simulink model "sm_trackV_test_frame_IdlerArm_i2u0r3"  (R2026a)
settings: Solver=VariableStepAuto  AbsTol=1e-3  EnableMultiTasking=on
undefined symbols (not defined in the file): Trac, X, Y, Z
libraries: sm_trackV_lib_belt_underc_elem x5, sm_lib x4, sm_trackV_lib_frame_idlerArm_i2u0l3 x1, nesl_utility x1
Description:
  | Copyright 2024-2026 The MathWorks, Inc.
settings Model: Creator=smiller  LastModifiedBy=smiller
settings DebuggingCC: SubsystemReferenceDiagnosticForUnitTest=warning
settings SimscapeCC: SimscapeNominalValues="[{\"value\":\"1\",\"unit\":\"A\"},{\"value\":\"1\",\"unit\":\"bar\"},{\"value\":\"1\",\"unit\":\"cm^2\"},{\"value\":\"1\",\"unit\":\"cm^3/s\"},{\"value\":\"1\",\"unit\":\"kJ/kg\"},{\"value\":\"1\",\"unit\":\"kW\"},{\"value\":\"1\",\"unit\":\"l\"},{\"value\":\"1\",\"unit\":\"N\"},{\"value\":\"1\",\"unit\":\"N*m\"},{\"value\":\"1\",\"unit\":\"V\"}]"  SimscapeLogSimulationStatistics=on
settings ExplorerConfigSet: InternalSimMechanicsExplorerSettings="<ExplorerConfiguration><canonicalview>default</canonicalview><AnimationSetting><BasePlaybackSpeed>1.0</BasePlaybackSpeed><PlaybackSpeedFactor>1.0</PlaybackSpeedFactor></AnimationSetting><TilePanel><TileInfo><Tiles Columns=\"1\" Count=\"1\" Rows=\"1\"><Column Weight=\"1\"/><Row Weight=\"1\"/><Tile Height=\"1\" Width=\"1\" X=\"0\" Y=\"0\"/></Tiles></TileInfo><SceneInfo><SceneViewer><BGColor><R>1</R><G>1</G><B>1</B></BGColor><Camera><DoPerspective>off</DoPerspective><Position><X>0.754785288464031145</X><Y>-1.88317428009450927</Y><Z>0.0238268327668960112</Z></Position><Center><X>-0.102012532308323189</X><Y>0.0261516749909807</Y><Z>-0.414185312493715541</Z></Center><Up><X>-0.0551998131405338766</X><Y>0.199660102991916943</Y><Z>0.97830916580726579</Z></Up><ViewLimDist>1</ViewLimDist><YLim>1.08093997579067946</YLim><XLim>1.28111404538154594</XLim></Camera></SceneViewer></SceneInfo></TilePanel><MechEditorPanel><Cameras/><GfxPanelCameraMap/><VideoCreator><PlaybackSpeedRatio>1.0</PlaybackSpeedRatio><FrameRate>30</FrameRate><VideoFormat>Motion JPEG AVI</VideoFormat><FrameSize>auto</FrameSize></VideoCreator></MechEditorPanel></ExplorerConfiguration>"

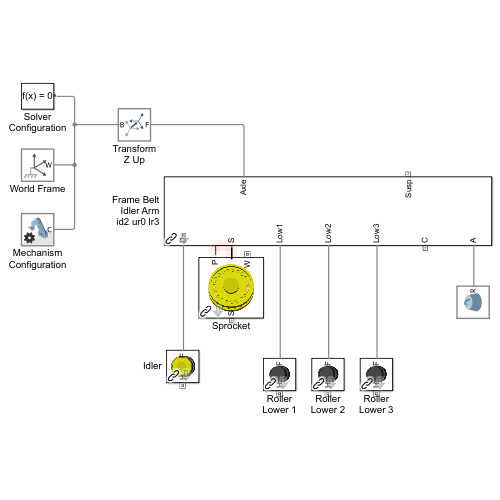
[thumbnail: Simulink's stored preview of the top-level diagram]
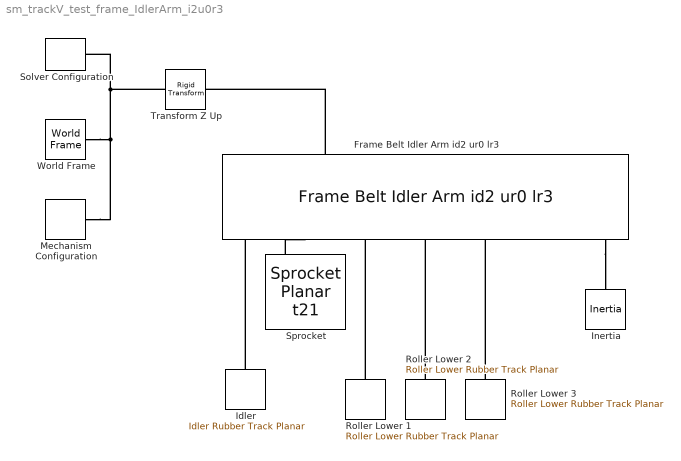
== system sm_trackV_test_frame_IdlerArm_i2u0r3 ==
  Frame Belt Idler Arm id2 ur0 lr3 : sm_trackV_lib_frame_idlerArm_i2u0l3/Frame Belt Idler Arm id2 ur0 lr3  popup_leftOrRight=Right  popup_trackFrame=Revolute  roller_lower_x=Trac.Frame.SprkOffLon.Lower  idlerArm_x=Trac.Frame.SprkOffLon.IdlerArm  idlerFix_x=Trac.Frame.SprkOffLon.IdlerR  tensionC_x=Trac.Frame.SprkOffLon.TensionC  frame_pivot_x=Trac.Frame.SprkOffLon.PivotFra  axle_x=Trac.Frame.SprkOffLon.Axle  roller_lower_y=Trac.Frame.SprkOffVer.Lower  idlerArm_y=Trac.Frame.SprkOffVer.IdlerArm  idlerFix_y=Trac.Frame.SprkOffVer.IdlerR  tensionC_y=Trac.Frame.SprkOffVer.TensionC  frame_pivot_y=Trac.Frame.SprkOffVer.PivotFra  axle_y=Trac.Frame.SprkOffVer.Axle  frame_roller_cg_offset=Trac.Frame.TrackFrame.CG  frame_roller_mass=Trac.Frame.TrackFrame.Mass  frame_roller_moi=Trac.Frame.TrackFrame.MOI  frame_roller_poi=Trac.Frame.TrackFrame.POI  frame_cg_offset=Trac.Frame.SprkFrame.CG  frame_mass=Trac.Frame.SprkFrame.Mass  frame_moi=Trac.Frame.SprkFrame.MOI  frame_poi=Trac.Frame.SprkFrame.POI  frame_susp_offset=Trac.Frame.SuspOffset  roller_frame_pivot_range=Trac.Frame.PivotFra.Range  roller_frame_pivot_k=Trac.Frame.PivotFra.LimitK  roller_frame_pivot_b=Trac.Frame.PivotFra.LimitB  roller_frame_pivot_tw=Trac.Frame.PivotFra.LimitTW
  Idler : sm_trackV_lib_belt_underc_elem/Idler Rubber Track Planar  idler_rad=Trac.IdlerF.rad  idler_len=Trac.IdlerF.len  wheel_clr=Trac.IdlerF.Wheel.clr  rim_rad=Trac.IdlerF.Rim.rad  rim_hub_rad=Trac.IdlerF.Rim.hub_rad  rim_xc=Trac.IdlerF.Rim.rim_xc  idler_rho=Trac.IdlerF.rho  idler_opc=Trac.IdlerF.opc  idler_clr=Trac.IdlerF.clr  idler_axle_rad=Trac.IdlerF.Axle.rad  idler_axle_len=Trac.IdlerF.Axle.len  idler_axle_rho=Trac.IdlerF.Axle.rho  idler_axle_opc=Trac.IdlerF.Axle.opc  idler_axle_clr=Trac.IdlerF.Axle.clr  idler_contgeo_clr=Trac.IdlerF.belt_contact.clr  idler_contgeo_opc=Trac.IdlerF.belt_contact.opc
  Inertia : sm_lib/Body Elements/Inertia  InertiaType=PointMass  Mass=1  MassUnits=kg  CenterOfMass=[0 0 0]  CenterOfMassUnits=m  MomentsOfInertia=[1 1 1]  MomentsOfInertiaUnits=kg*m^2  ProductsOfInertia=[0 0 0]  ProductsOfInertiaUnits=kg*m^2  GraphicType=Marker  MarkerShape=Inertia  MarkerSize=20  GraphicVisPropType=SimpleVisualProperties  GraphicDiffuseColor=[0.5 0.5 0.5]  GraphicOpacity=1.0  GraphicSpecularColor=[0.5 0.5 0.5 1.0]  GraphicAmbientColor=[0.15 0.15 0.15 1.0]  GraphicEmissiveColor=[0.0 0.0 0.0 1.0]  GraphicShininess=75
  Mechanism Configuration : sm_lib/Utilities/Mechanism Configuration  UniformGravity=Constant  GravityVector=[0 0 -9.80665]  GravityVectorUnits=m/s^2  LinearizationDelta=0.001  JointModeTransitionNonlinearIterations=2
  Roller Lower 1 : sm_trackV_lib_belt_underc_elem/Roller Lower Rubber Track Planar  roller_lower_rad=Trac.Roller.Lower.rad  roller_lower_len=Trac.Roller.Lower.len  roller_lower_rho=Trac.Roller.Lower.rho  roller_lower_clr=Trac.Roller.Lower.clr  roller_lower_opc=Trac.Roller.Lower.opc  roller_lower_rim_thk=Trac.Roller.Lower.rim_thk  roller_lower_rim_len=Trac.Roller.Lower.rim_len  roller_lower_axle_rad=Trac.Roller.Lower.Axle.rad  roller_lower_axle_len=Trac.Roller.Lower.Axle.len  roller_lower_axle_rho=Trac.Roller.Lower.Axle.rho  roller_lower_axle_opc=Trac.Roller.Lower.Axle.opc  roller_lower_axle_clr=Trac.Roller.Lower.Axle.clr  roller_lower_contgeo_clr=Trac.Roller.Lower.belt_contact.ptcld.clr  roller_lower_contgeo_opc=Trac.Roller.Lower.belt_contact.ptcld.opc
  Roller Lower 2 : sm_trackV_lib_belt_underc_elem/Roller Lower Rubber Track Planar  roller_lower_rad=Trac.Roller.Lower.rad  roller_lower_len=Trac.Roller.Lower.len  roller_lower_rho=Trac.Roller.Lower.rho  roller_lower_clr=Trac.Roller.Lower.clr  roller_lower_opc=Trac.Roller.Lower.opc  roller_lower_rim_thk=Trac.Roller.Lower.rim_thk  roller_lower_rim_len=Trac.Roller.Lower.rim_len  roller_lower_axle_rad=Trac.Roller.Lower.Axle.rad  roller_lower_axle_len=Trac.Roller.Lower.Axle.len  roller_lower_axle_rho=Trac.Roller.Lower.Axle.rho  roller_lower_axle_opc=Trac.Roller.Lower.Axle.opc  roller_lower_axle_clr=Trac.Roller.Lower.Axle.clr  roller_lower_contgeo_clr=Trac.Roller.Lower.belt_contact.ptcld.clr  roller_lower_contgeo_opc=Trac.Roller.Lower.belt_contact.ptcld.opc
  Roller Lower 3 : sm_trackV_lib_belt_underc_elem/Roller Lower Rubber Track Planar  roller_lower_rad=Trac.Roller.Lower.rad  roller_lower_len=Trac.Roller.Lower.len  roller_lower_rho=Trac.Roller.Lower.rho  roller_lower_clr=Trac.Roller.Lower.clr  roller_lower_opc=Trac.Roller.Lower.opc  roller_lower_rim_thk=Trac.Roller.Lower.rim_thk  roller_lower_rim_len=Trac.Roller.Lower.rim_len  roller_lower_axle_rad=Trac.Roller.Lower.Axle.rad  roller_lower_axle_len=Trac.Roller.Lower.Axle.len  roller_lower_axle_rho=Trac.Roller.Lower.Axle.rho  roller_lower_axle_opc=Trac.Roller.Lower.Axle.opc  roller_lower_axle_clr=Trac.Roller.Lower.Axle.clr  roller_lower_contgeo_clr=Trac.Roller.Lower.belt_contact.ptcld.clr  roller_lower_contgeo_opc=Trac.Roller.Lower.belt_contact.ptcld.opc
  Solver Configuration : nesl_utility/Solver Configuration  PhysicalDomain=network_engine_domain  SubClassName=solver  LeftPortType=input  RightPortType=generic  Tones=[]  Harmonics=[]  SimulateNoise=off  Profile=off  UseLocalSampling=off  EnableSwitchedLinearOptims=on  FrequencyDomain=off  UseCCode=off  RelTol=0.001  AbsTol=1e-06  MinStep=1e-09  ToWorkspace=off  RevertToSquareIcSolve=off  NumHomotopyIterations=100  PhasorMode=off  PhasorModeNumHarmonics=1  ConsistencySolver=NEWTON_XTOL_AFTER_FTOL  CanonicalOrdering=UNORDERED  OptimizeIntermediates=UNOPTIMIZED  IndexReductionMethod=DerivativeReplacement  DoDC=off  ResidualTolerance=1e-09  ConsistencyTolSource=GLOBAL  ConsistencyAbsTol=0.001  ConsistencyRelTol=0.001  ConsistencyTolFactor=0.001  UseLocalSolver=off  LocalSolverChoice=NE_BACKWARD_EULER_ADVANCER  ResolveIndetEquations=on  FunctionEvalNumThread=1  LocalSolverSampleTime=0.001  DoFixedCost=off  MaxNonlinIter=3  MaxModeIter=2  ComputeImpulses=off  ImpulseIterations=2  LinearAlgebra=Sparse  LinearAlgebraNumThread=0  EquationFormulation=NE_TIME_EF  DelaysMemoryBudget=1024  AutomaticFiltering=on  FilteringTimeConstant=0.001  PartitionStorageMethod=AS_NEEDED  PartitionMemoryBudget=1024  PartitionMethod=FAST  MultibodyUseLocalSolver=off  MultibodyLocalSolverChoice=ODE1  MultibodyLocalSolverSampleTime=0.001
  Sprocket : sm_trackV_lib_belt_underc_elem/Sprocket Planar t21  sprk_wid_roll=Trac.Sprocket.Roller.wid  sprk_rad_roll=Trac.Sprocket.Roller.rad  sprk_opc=Trac.Sprocket.Roller.opc*0.5  sprk_clr=Trac.Sprocket.Roller.clr  sprk_rad_pitch=Trac.Sprocket.Pin.pitch_rad  sprk_spoke_rad=Trac.Sprocket.Spoke.rad  sprk_spoke_len=Trac.Sprocket.Spoke.len  sprk_spoke_num=Trac.Sprocket.nSpokes  sprk_spoke_clr=Trac.Sprocket.Spoke.clr  sprk_spoke_opc=Trac.Sprocket.Spoke.opc  rim_spoke_xc=Trac.Sprocket.Rim.spoke_xc  rim_thk=Trac.Sprocket.Rim.thk  rim_ir=Trac.Sprocket.Rim.rad_inner  sprk_contgeo_roller_clr=Trac.Sprocket.roller_contact.clr  sprk_contgeo_roller_opc=Trac.Sprocket.roller_contact.opc  sprk_contgeo_spoke_clr=Trac.Sprocket.spoke_contact.clr  sprk_contgeo_spoke_opc=Trac.Sprocket.spoke_contact.opc
  Transform Z Up : sm_lib/Frames and Transforms/Rigid Transform  RotationMethod=StandardAxis  FollAlignAxisA=+X  BaseAlignAxisA=+Y  FollAlignAxisB=+Y  BaseAlignAxisB=+Z  RotationStandardAxis=+X  RotationAngle=-90  RotationAngleUnits=deg  RotationArbitraryAxis=[0 0 1]  RotationSequenceAxes=FollowerAxes  RotationSequence=XYX  RotationSequenceAngles=[0 0 0]  RotationSequenceAnglesUnits=deg  RotationMatrix=[1 0 0; 0 1 0; 0 0 1]  Quaternion=[1 0 0 0]  TranslationMethod=None  TranslationCartesianOffset=[0 0 0]  TranslationCartesianOffsetUnits=m  TranslationStandardAxis=+Z  TranslationStandardOffset=0  TranslationStandardOffsetUnits=m  TranslationROffset=0  TranslationROffsetUnits=m  TranslationThetaOffset=0  TranslationThetaOffsetUnits=deg  TranslationZOffset=0  TranslationZOffsetUnits=m
  World Frame : sm_lib/Frames and Transforms/World Frame
  connections:
  World Frame/RConn1 -- Transform Z Up/LConn1 -- Solver Configuration/RConn1 -- Mechanism Configuration/RConn1
  Frame Belt Idler Arm id2 ur0 lr3/RConn1 -- Inertia/RConn1
  Sprocket/LConn1 -- Frame Belt Idler Arm id2 ur0 lr3/RConn6
  Roller Lower 1/LConn1 -- Frame Belt Idler Arm id2 ur0 lr3/RConn5
  Roller Lower 2/LConn1 -- Frame Belt Idler Arm id2 ur0 lr3/RConn4
  Roller Lower 3/LConn1 -- Frame Belt Idler Arm id2 ur0 lr3/RConn3
  Idler/LConn1 -- Frame Belt Idler Arm id2 ur0 lr3/RConn7
  Frame Belt Idler Arm id2 ur0 lr3/LConn2 -- Transform Z Up/RConn1
